simulink model "vipliveedgedetection_win"  (R2015b)
settings: Solver=FixedStepDiscrete  StartTime=0.0  StopTime=inf  RelTol=1e-3
undefined symbols (not defined in the file or in its folder): EdgeTrigger, FallingEdge, videoinput
libraries: visionsinks x3, visiontextngfix x1, visionanalysis x1, imaqlib x1, vipmisc x1
settings Model: FPTRunName=Active  ExtModeAutoUpdateStatusClock=off  Creator=The MathWorks, Inc.  LastModifiedBy=The MathWorks, Inc.
settings DataIOCC: LimitDataPoints=off  SaveFormat=Array  SaveOutput=off  SaveTime=off  SignalLoggingName=sigsOut
settings OptimizationCC: ExpressionDepthLimit=2147483647  InitFltsAndDblsToZero=on
settings DebuggingCC: UnderspecifiedInitializationDetection=Classic  MergeDetectMultiDrivingBlocksExec=none  CheckExecutionContextPreStartOutputMsg=on  CheckExecutionContextRuntimeOutputMsg=on  SignalResolutionControl=TryResolveAllWithWarning  MultiTaskDSMMsg=warning  MultiTaskCondExecSysMsg=none  SigSpecEnsureSampleTimeMsg=none  FcnCallInpInsideContextMsg=UseLocalSettings  StateNameClashWarn=warning  StrictBusMsg=None
settings HardwareCC: ProdBitPerPointer=32  ProdLargestAtomicFloat=None  ProdIntDivRoundTo=Undefined  ProdEndianess=Unspecified  ProdWordSize=32  ProdHWDeviceType=32-bit Generic  TargetBitPerLong=64  TargetBitPerPointer=64  TargetLongLongMode=on  TargetIntDivRoundTo=Zero  TargetEndianess=LittleEndian  TargetWordSize=64  TargetHWDeviceType=Generic->MATLAB Host Computer  ProdEqTarget=off
settings GRTTargetCC: TargetFcnLib=ansi_tfl_tmw_new.mat  GeneratePreprocessorConditionals=Disable all  CombineOutputUpdateFcns=off  GRTInterface=on
settings ConfigComp: CovModelRefEnable=Off

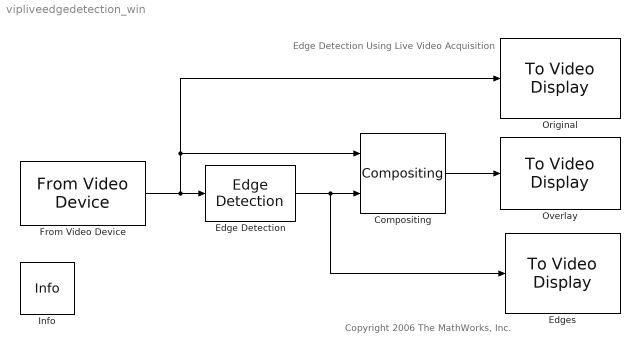
== system vipliveedgedetection_win ==
  note: Edge Detection Using Live Video Acquisition
  note: Copyright 2006 The MathWorks, Inc.
  Compositing : visiontextngfix/Compositing  operation=Highlight selected pixels  bFacSrc=Input port  mFacSrc=Input port  bFactor=0.75  mFactor=1  source=Specify via dialog  coordinates=[1 1]  prodOutputMode=Binary point scaling  prodOutputWordLength=32  prodOutputFracLength=10  roundingMode=Floor  overflowMode=off
  Edge Detection : visionanalysis/Edge Detection  method=Prewitt  outputType=Binary image  userDefinedThreshold=on  thresholdSource=Specify via dialog  threshold=single(15/256)  thresholdTuning=4  edgeThinning=on  threshold_canny=[0.25 0.60]  autoPercent=70  sigma=1  roundingMode=Floor  overflowMode=off
  Edges : visionsinks/To Video Display  windowSizeMode=True size (1:1)  openAtMdlStart=on  fullScreen=off  videoWindowX=444  videoWindowY=313  saveWindowSize=off  videoWindowWidth=168  videoWindowHeight=147  inputColorFormat=RGB  inputType=Obsolete  imagePorts=One multidimensional signal  OutputDevice=On-screen video monitor  dataOrg=Column-major  isWindowOpen=off
  From Video Device : imaqlib/From Video Device  DeviceMenu=demo 1 (Color Device)  Device="hamamatsu 1 (Hamamatsu 1394 C8484-05G  S/N: 750135  Bus: OHCI 1394)"  ObjConstructor=videoinput('hamamatsu', 1)  VideoFormatMenu=RGB_NTSC  VideoFormat=MONO8_BIN4x4_336x256  VideoSource=input1  ROIPosition=[0 0 256 336]  EnableHWTrigger=off  TriggerConfiguration=EdgeTrigger/FallingEdge  SampleTime=1/30  OutputPortsMode=One multidimensional signal  DataType=single  CanDoHWTrigger=yes  ReturnedColorSpace=grayscale  BlockHandle=30.1971  ROIWidth=336  ROIHeight=256  ROIColumn=0  ROIRow=0  EngXMLPath=/mathworks/devel/bat/BR2015bd/build/matlab/toolbox/imaq/imaq/private  DevXMLPath=/mathworks/devel/bat/BR2015bd/build/matlab/toolbox/imaq/imaqadaptors/glnxa64  EngLibPath=/mathworks/devel/bat/BR2015bd/build/matlab/toolbox/imaq/imaqblks/imaqmex/glnxa64  ColorSpace=rgb  BayerSensorAlignment=grbg
  Info : vipmisc/Info  SystemSampleTime=-1
  Original : visionsinks/To Video Display  windowSizeMode=True size (1:1)  openAtMdlStart=on  fullScreen=off  videoWindowX=100  videoWindowY=312  saveWindowSize=off  videoWindowWidth=168  videoWindowHeight=147  inputColorFormat=RGB  inputType=Obsolete  imagePorts=One multidimensional signal  OutputDevice=On-screen video monitor  dataOrg=Column-major  isWindowOpen=off
  Overlay : visionsinks/To Video Display  windowSizeMode=True size (1:1)  openAtMdlStart=on  fullScreen=off  videoWindowX=787  videoWindowY=313  saveWindowSize=off  videoWindowWidth=168  videoWindowHeight=147  inputColorFormat=RGB  inputType=Obsolete  imagePorts=One multidimensional signal  OutputDevice=On-screen video monitor  dataOrg=Column-major  isWindowOpen=off
  wires:
  From Video Device/1 -> Edge Detection/1, Original/1, Compositing/1
  Compositing/1 -> Overlay/1
  Edge Detection/1 -> Edges/1, Compositing/2
